simulink model "test_pid_pd_regler_2"  (R2016b)
settings: Solver=FixedStepAuto  StartTime=0.0  StopTime=50.0  FixedStep=1e-3  RelTol=1e-3
undefined symbols (not defined in the file or in its folder): param
libraries: simulink x3, simulink_extras x2
settings Model: Creator=nicol  LastModifiedBy=Fritz

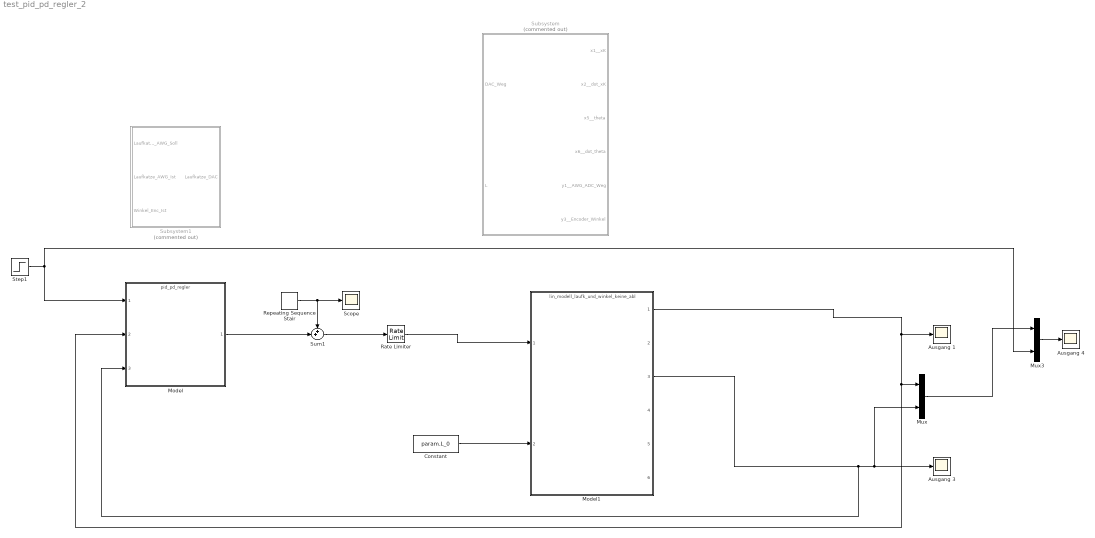
== system test_pid_pd_regler_2 ==
  Ausgang 1 : Scope
  Ausgang 3 : Scope
  Ausgang 4 : Scope
  Constant : Constant  Value=param.L_0
  Model : ModelReference  ModelNameDialog=pid_pd_regler.slx  SimulationMode=Normal  ModelReferenceVersion=1.8
  Model1 : ModelReference  ModelNameDialog=lin_modell_laufk_und_winkel_keine_abl.slx  SimulationMode=Normal  ModelReferenceVersion=1.37
  Mux : Mux  Inputs=2
  Mux3 : Mux  Inputs=2
  Rate Limiter : RateLimiter  RisingSlewLimit=4.32  FallingSlewLimit=-4.32  SampleTimeMode=inherited
  Repeating Sequence Stair : simulink/Sources/Repeating Sequence Stair  OutValues=[0.2 0.3]  tsamp=1  OutMin=[]  OutMax=[]  OutDataTypeStr=double  OutputDataTypeScalingMode=double  OutDataType=fixdt(0,8)  ConRadixGroup=Best Precision: Vector-wise  OutScaling=2^-12
  Scope : Scope
  Step1 : Step  SampleTime=0
  Subsystem : Subsystem  Commented=on
  Subsystem1 : Subsystem  Commented=on
  Sum1 : Sum  Inputs=++|
  wires:
  Mux/1 -> Mux3/1
  Mux3/1 -> Ausgang 4/1
  Step1/1 -> Model/1, Mux3/2
  Repeating Sequence Stair/1 -> Scope/1, Sum1/1
  Sum1/1 -> Rate Limiter/1
  Model1/1 -> Model/2, Mux/1, Ausgang 1/1
  Model1/3 -> Model/3, Mux/2, Ausgang 3/1
  Rate Limiter/1 -> Model1/1
  Constant/1 -> Model1/2
  Model/1 -> Sum1/2

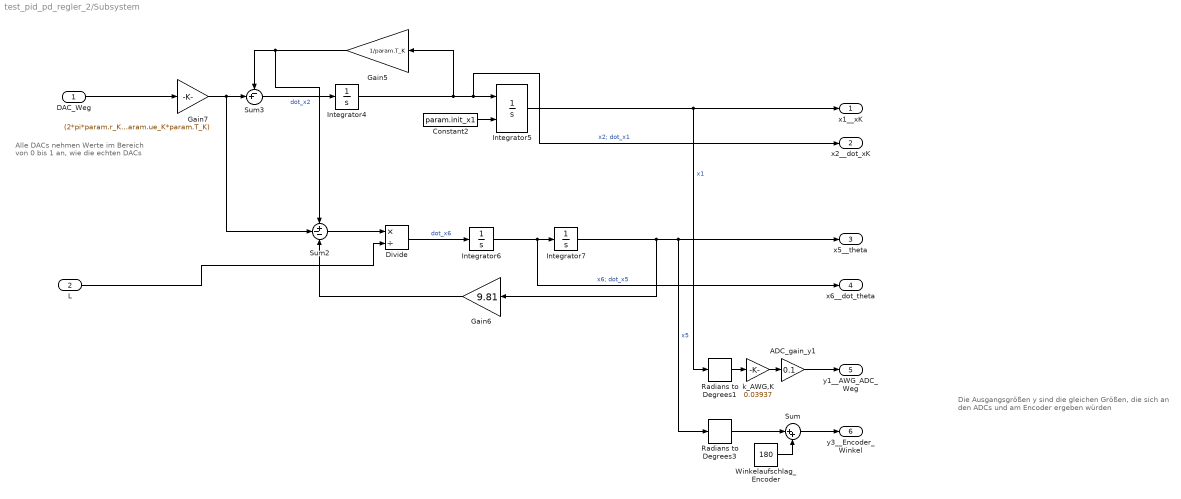
== system test_pid_pd_regler_2/Subsystem ==
  note: Die Ausgangsgrößen y sind die gleichen Größen,
      | die sich an den ADCs und am Encoder ergeben würden
  note: Alle DACs nehmen Werte im Bereich
      | von 0 bis 1 an, wie die echten DACs
  DAC_Weg : Inport
  L : Inport  Port=2
  ADC_gain_y1 : Gain  Gain=0.1
  Constant2 : Constant  Value=param.init_x1
  Divide : Product  Inputs=*/
  Gain5 : Gain  Gain=1/param.T_K
  Gain6 : Gain  Gain=9.81
  Gain7 : Gain  Gain=(2*pi*param.r_K*param.K_K)/(param.ue_K*param.T_K)
  Integrator4 : Integrator
  Integrator5 : Integrator  InitialConditionSource=external
  Integrator6 : Integrator
  Integrator7 : Integrator
  Radians to Degrees1 : simulink_extras/Transformations/Radians to Degrees
  Radians to Degrees3 : simulink_extras/Transformations/Radians to Degrees
  Sum : Sum  Inputs=|++
  Sum2 : Sum  Inputs=+--
  Sum3 : Sum  Inputs=-+|
  Winkelaufschlag_Encoder : Constant  Value=180
  k_AWG,K : Gain  Gain=0.03937
  x1__xK : Outport
  x2__dot_xK : Outport  Port=2
  x5__theta : Outport  Port=3
  x6__dot_theta : Outport  Port=4
  y1__AWG_ADC_Weg : Outport  Port=5
  y3__Encoder_Winkel : Outport  Port=6
  wires:
  k_AWG,K/1 -> ADC_gain_y1/1
  Winkelaufschlag_Encoder/1 -> Sum/2
  Sum/1 -> y3__Encoder_Winkel/1
  ADC_gain_y1/1 -> y1__AWG_ADC_Weg/1
  DAC_Weg/1 -> Gain7/1
  Sum3/1 -> Integrator4/1  "dot_x2"
  Integrator4/1 -> x2__dot_xK/1, Integrator5/1, Gain5/1  "x2; dot_x1"
  Gain5/1 -> Sum2/1, Sum3/1
  Constant2/1 -> Integrator5/2
  Gain7/1 -> Sum2/2, Sum3/2
  Sum2/1 -> Divide/1
  Divide/1 -> Integrator6/1  "dot_x6"
  Integrator6/1 -> x6__dot_theta/1, Integrator7/1  "x6; dot_x5"
  Integrator7/1 -> x5__theta/1, Radians to Degrees3/1, Gain6/1  "x5"
  Gain6/1 -> Sum2/3
  Integrator5/1 -> Radians to Degrees1/1, x1__xK/1  "x1"
  L/1 -> Divide/2
  Radians to Degrees1/1 -> k_AWG,K/1
  Radians to Degrees3/1 -> Sum/1

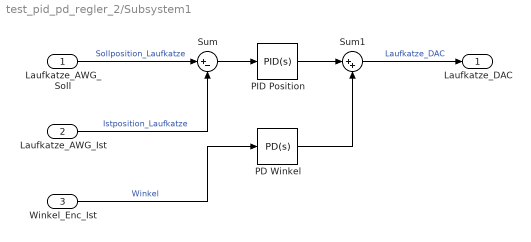
== system test_pid_pd_regler_2/Subsystem1 ==
  Laufkatze_AWG_Soll : Inport
  Laufkatze_AWG_Ist : Inport  Port=2
  Winkel_Enc_Ist : Inport  Port=3
  PD Winkel : simulink/Continuous/PID Controller  Controller=PD  TimeDomain=Continuous-time  SampleTime=-1  IntegratorMethod=Forward Euler  FilterMethod=Forward Euler  Form=Parallel  UseFilter=on  ControllerParametersSource=internal  P=50  I=0  D=10  N=100  InitialConditionSource=internal  InitialConditionForIntegrator=0  InitialConditionForFilter=0  ExternalReset=none  LimitOutput=off  UpperSaturationLimit=inf  LowerSaturationLimit=-inf  LinearizeAsGain=on  AntiWindupMode=none  Kb=1  TrackingMode=off  Kt=1  PParamMin=[]  PParamMax=[]  IParamMin=[]  IParamMax=[]  DParamMin=[]  DParamMax=[]  NParamMin=[]  NParamMax=[]  KbParamMin=[]  KbParamMax=[]  KtParamMin=[]  KtParamMax=[]  POutMin=[]  POutMax=[]  IOutMin=[]  IOutMax=[]  DOutMin=[]  DOutMax=[]  NOutMin=[]  NOutMax=[]  KbOutMin=[]  KbOutMax=[]  KtOutMin=[]  KtOutMax=[]  IntegratorOutMin=[]  IntegratorOutMax=[]  FilterOutMin=[]  FilterOutMax=[]  SumOutMin=[]  SumOutMax=[]  SumI1OutMin=[]  SumI1OutMax=[]  SumI2OutMin=[]  SumI2OutMax=[]  SumI3OutMin=[]  SumI3OutMax=[]  SumDOutMin=[]  SumDOutMax=[]  SaturationOutMin=[]  SaturationOutMax=[]  IntegratorContinuousStateAttributes=''  IntegratorStateMustResolveToSignalObject=off  IntegratorRTWStateStorageClass=Auto  FilterContinuousStateAttributes=''  FilterStateMustResolveToSignalObject=off  FilterRTWStateStorageClass=Auto  DifferentiatorICPrevScaledInput=0  DifferentiatorOutMin=[]  DifferentiatorOutMax=[]
  PID Position : simulink/Continuous/PID Controller  Controller=PID  TimeDomain=Continuous-time  SampleTime=-1  IntegratorMethod=Forward Euler  FilterMethod=Forward Euler  Form=Parallel  UseFilter=on  ControllerParametersSource=internal  P=40  I=3  D=1  N=100  InitialConditionSource=internal  InitialConditionForIntegrator=0  InitialConditionForFilter=0  ExternalReset=none  LimitOutput=off  UpperSaturationLimit=inf  LowerSaturationLimit=-inf  LinearizeAsGain=on  AntiWindupMode=none  Kb=1  TrackingMode=off  Kt=1  PParamMin=[]  PParamMax=[]  IParamMin=[]  IParamMax=[]  DParamMin=[]  DParamMax=[]  NParamMin=[]  NParamMax=[]  KbParamMin=[]  KbParamMax=[]  KtParamMin=[]  KtParamMax=[]  POutMin=[]  POutMax=[]  IOutMin=[]  IOutMax=[]  DOutMin=[]  DOutMax=[]  NOutMin=[]  NOutMax=[]  KbOutMin=[]  KbOutMax=[]  KtOutMin=[]  KtOutMax=[]  IntegratorOutMin=[]  IntegratorOutMax=[]  FilterOutMin=[]  FilterOutMax=[]  SumOutMin=[]  SumOutMax=[]  SumI1OutMin=[]  SumI1OutMax=[]  SumI2OutMin=[]  SumI2OutMax=[]  SumI3OutMin=[]  SumI3OutMax=[]  SumDOutMin=[]  SumDOutMax=[]  SaturationOutMin=[]  SaturationOutMax=[]  IntegratorContinuousStateAttributes=''  IntegratorStateMustResolveToSignalObject=off  IntegratorRTWStateStorageClass=Auto  FilterContinuousStateAttributes=''  FilterStateMustResolveToSignalObject=off  FilterRTWStateStorageClass=Auto  DifferentiatorICPrevScaledInput=0  DifferentiatorOutMin=[]  DifferentiatorOutMax=[]
  Sum : Sum  Inputs=|+-
  Sum1 : Sum  Inputs=|++
  Laufkatze_DAC : Outport
  wires:
  Laufkatze_AWG_Soll/1 -> Sum/1  "Sollposition_Laufkatze"
  Laufkatze_AWG_Ist/1 -> Sum/2  "Istposition_Laufkatze"
  Sum/1 -> PID Position/1
  PID Position/1 -> Sum1/1
  Winkel_Enc_Ist/1 -> PD Winkel/1  "Winkel"
  PD Winkel/1 -> Sum1/2
  Sum1/1 -> Laufkatze_DAC/1  "Laufkatze_DAC"
